simulink model "DDSM"  (R2020b)
settings: Solver=VariableStepAuto  StartTime=0.0  StopTime=1000.0  RelTol=1e-3
libraries: dspstat3 x1
settings Model: Creator=chank  LastModifiedBy=chank

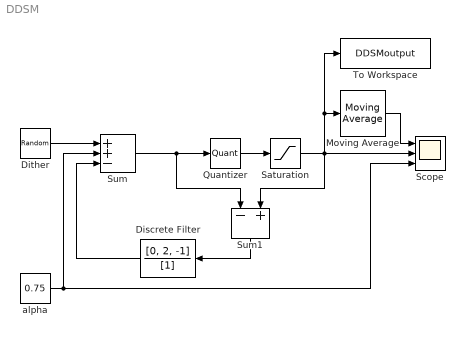
== system DDSM ==
  Discrete Filter : DiscreteFilter  Numerator=[0, 2, -1]  Denominator=[1]
  Dither : RandomNumber  SampleTime=0.1
  Moving Average : dspstat3/Moving Average  Method=Sliding window  ForgettingFactorPort=off  SpecifyWindowLength=on  WindowLength=100  ForgettingFactor=0.9  SimulateUsing=Code generation
  Quantizer : Quantizer  QuantizationInterval=1
  Saturation : Saturate  UpperLimit=2  LowerLimit=-2
  Scope : Scope  NumInputPorts=3
  Sum : Sum  Inputs=|+|+|-|
  Sum1 : Sum  Inputs=-|+
  To Workspace : ToWorkspace  VariableName=DDSMoutput  SaveFormat=Timeseries  SampleTime=-1
  alpha : Constant  Value=0.75
  wires:
  Quantizer/1 -> Saturation/1
  Dither/1 -> Sum/1
  alpha/1 -> Scope/3, Sum/2
  Sum/1 -> Quantizer/1, Sum1/1
  Saturation/1 -> To Workspace/1, Moving Average/1, Scope/2, Sum1/2
  Sum1/1 -> Discrete Filter/1
  Discrete Filter/1 -> Sum/3
  Moving Average/1 -> Scope/1
